simulink model "prova_kalman_09_28_BUONO"  (R2020b)
settings: Solver=ode4  StartTime=0.0  StopTime=Inf  FixedStep=0.02  RelTol=1e-3
PostLoadFcn:
  | , if any(exist('dsrtsu_mdlpostloadfcn', 'file') == [2, 3, 6]), try dsrtsu_mdlpostloadfcn('Execute', bdroot); catch fprintf('Error in PostLoadFcn (dsrtsu_mdlpostloadfcn) for model "%s":\n %s\n', bdroot, lasterr); end, end,
InitFcn:
  | , if any(exist('rtifpga_mdlclblib', 'file') ~= 0), rtifpga_mdlclblib('Init', bdroot); end,
values from neighbouring files (symbols this model uses):
  bias = [baccxINI_new,baccyINI_new,bacczINI_new,bpINI_new,bqINI_new,brINI_new]    [Loader_volo.m]
  Q1B = [    2e-15;                  2e-15 ... (first row only)    [COV_F1B_HIL.m]    (also in COV_F1B_VOLO_UP1.m = [    1.4e-14;                  1.5e-14; COV_F1B_VOLO_UP2.m = [    1.2e-14;                  1.7e-14)
  R1B = [     2e-14;                   2e-14 ... (first row only)    [COV_F1B_HIL.m]    (also in COV_F1B_VOLO_UP1.m = [     1e-13;                  1e-13; COV_F1B_VOLO_UP2.m = [     0.75e-13;                  0.9e-13)
  Sensor_Offsets = [0,0,0]    [Loader_volo.m]
  T_cal = 0.4    [Loader_volo.m]
  UP = 1    [Loader_volo.m]
  vd_ini = 0    [Loader_volo.m]
undefined symbols (not defined in the file or in its folder): DiscIntNeverNeededParam, Green, led0
libraries: simulink_extras x12, embdlinuxlib x3, raspberrypiCommlib x2, svdutilitieslib x2, aerosimlib x2, raspberrypiBasiclib x1, dspsigops x1
Description:
  | Standard RTI1006 template.
  | Supported MATLAB version:  R2020b.
settings Model: Tag=RTI1006  DSRTSU_INTERNAL_RTI_VER=570  DSRTSU_INTERNAL_RTI_TYPE=rti1006  RTICANMMDATA=struct('GeneralSetupData',struct('modelroot','C:\SUBTEAMS_2020_2021\SOFTWARE\AUTOPILOTA\drive1\Load_hardware\Raspberry_v2_1','generalsettings',struct('filesettings',struct('destfolder',struct('Name','RTICANMM_FILES','Check',1),'buildfolder',struct('Name','.','Check',1),'AbsDestfolder',struct('Name','C:\SUBTEAMS_2020_2021\SOFTWARE\AUTOPILOTA\drive1\Load_hardware\Raspberry_v2_1\RTICANMM_FILES'),'AbsBuildfolder',struct('Name','C:\SUBTEAMS_2020_2021\SOFTWARE\AUTOPILOTA\drive1\Load_hardware\Raspberry_v2_1'))),'options',struct('addpaths',1,'rmpaths',1,'addtrcexclusion',true,'cannavigator',struct('checkmonitoring',0),'show_usrtrc',0,'use_usrtrc',0),'advanced',struct('options',ones(1,100)),'MPSetup',{{}},'RTI',struct('Type','ERT','Ver','','Date',''),'modelname','prova_kalman_09_28_BUONO','block','prova_kalman_09_28_BUONO'))  DSRTSU_INTERNAL_RTIFPGA=170  Creator=lapis-dspace  LastModifiedBy=lapis-dspace
settings SolverCC: PositivePriorityOrder=on
settings DataIOCC: SaveOutput=off  SignalLogging=off  DSMLogging=off  SaveTime=off  ReturnWorkspaceOutputs=off
settings OptimizationCC: EnhancedBackFolding=on  PassReuseOutputArgsAs=Individual arguments  MaxStackSize=64  OptimizeBlockOrder=speed  DifferentSizesBufferReuse=on  OptimizationCustomize=off  EfficientTunableParamExpr=on
settings DebuggingCC: ParameterTunabilityLossMsg=error  PregeneratedLibrarySubsystemCodeDiagnostic=none  ArithmeticOperatorsInVariantConditions=warning
settings HardwareCC: ProdBitPerPointer=32  ProdBitPerSizeT=32  ProdBitPerPtrDiffT=32  ProdLargestAtomicInteger=Long  ProdLargestAtomicFloat=Double  ProdWordSize=32  ProdHWDeviceType=ARM Compatible->ARM Cortex  TargetIntDivRoundTo=Zero  TargetEndianess=LittleEndian  TargetHWDeviceType=Custom Processor->Custom
settings SFSimCC: SimUseLocalCustomCode=off  MATLABDynamicMemAlloc=off  CustomCodeUndefinedFunction=UseInterfaceOnly
settings RTWCC: Description=Embedded Coder  SystemTargetFile=ert.tlc  HardwareBoard=Raspberry Pi  TLCOptions="-aInlineSetEventsForThisBaseRateFcn=TLC_FALSE -aSuppressMultiTaskScheduler=TLC_FALSE  -aRateBasedStepFcn=0"  TemplateMakefile=ert_default_tmf  RTWUseLocalCustomCode=off  Toolchain=GNU GCC Raspberry Pi  BuildConfiguration=Faster Runs
settings CodeAppCC: ForceParamTrailComments=on  IgnoreCustomStorageClasses=off  OperatorAnnotations=on  SimulinkDataObjDesc=on  SFDataObjDesc=on  InsertBlockDesc=on
settings ERTTargetCC: MatFileLogging=on  SupportVariableSizeSignals=on
settings ConfigComp: CovMetricSettings=dswe

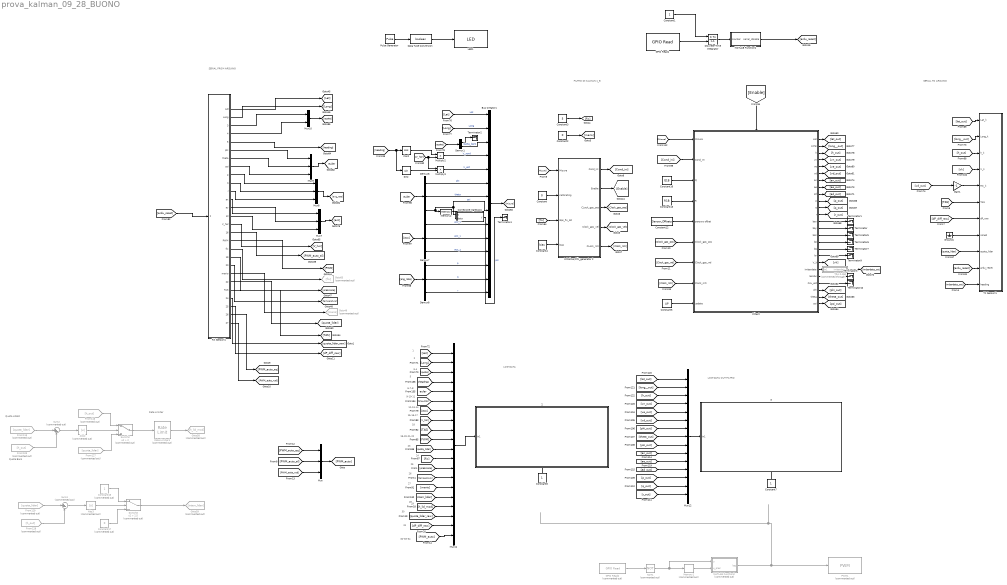
== system prova_kalman_09_28_BUONO ==
  note: 32-33-34
  note: 31
  note: 30
  note: 29
  note: 28
  note: 27
  note: 26
  note: 25
  note: 24
  note: 23
  note: 19-20-21-22
  note: 18
  note: 15-16-17
  note: 12-13-14
  note: 9-10-11
  note: 6-7-8
  note: 5
  note: 3-4
  note: 1
  note: SERIAL FROM ARDUINO
  note: LOG-DATA
  note: SERIAL TO ARDUINO
  note: LOG-DATA OUT FILTRO
  note: FILTRO DI KALMAN 1_B
  note: Rate Limiter
  note: Quota Baro
  note: Quota LIDAR
  note: 2
  " 2" : Subsystem
  " 3" : Subsystem
  Abs2 : Abs  Commented=on
  Abs3 : Abs  Commented=on
  Bus Creator1 : BusCreator  Inputs=14
  Constant : Constant  Value=0
  Constant1 : Constant  SampleTime=0.02
  Constant12 : Constant  Value=Sensor_Offsets
  Constant13 : Constant  Value=R1B
  Constant15 : Constant  Commented=on
  Constant16 : Constant  Value=Q1B
  Constant17 : Constant  Commented=on  Value=0
  Constant2 : Constant  Value=0
  Constant3 : Constant  Value=5
  Constant4 : Constant  Value=bias
  Constant5 : Constant  Value=UP
  Constant6 : Constant
  Constant7 : Constant
  Correzione ingresso1 : MATLAB Function  TreatAsAtomicUnit=on
  Cos2 : Trigonometry  Operator=cos
  Data Type Conversion : DataTypeConversion  OutDataTypeStr=boolean
  Demux1 : Demux  Outputs=2
  Demux6 : Demux  Outputs=3
  Demux7 : Demux  Outputs=3
  Demux8 : Demux  Outputs=3
  Discrete-Time Integrator : DiscreteIntegrator  ExternalReset=falling  SampleTime=0.02  LimitOutput=on  UpperSaturationLimit=1  LowerSaturationLimit=0  ICPrevOutput=DiscIntNeverNeededParam  ICPrevScaledInput=DiscIntNeverNeededParam
  Filter2 : Subsystem
  From103 : From  Commented=on  GotoTag=h_out
  From113 : From  Commented=on  GotoTag=quota_lidar
  From116 : From  Commented=on  GotoTag=h_out
  From127 : From  Commented=on  GotoTag=quota_lidar
  From128 : From  Commented=on  GotoTag=h_out
  From129 : From  Commented=on  GotoTag=quota_lidar
  GPIO Read1 : embdlinuxlib/GPIO Read  board=Pi 3 Model B  gpio=21  internalResistor=Off  sampleTime=0.02  direction=Input  blockPlatform=Raspberry Pi
      settings: SourceProductBaseCode=SC_BEAGLEBONE_BLUE,NVIDIA,RASPPI
  GPIO Read2 : embdlinuxlib/GPIO Read  Commented=on  board=Pi 3 Model B  gpio=4  internalResistor=Off  sampleTime=0.1  direction=Input  blockPlatform=Raspberry Pi
      settings: SourceProductBaseCode=SC_BEAGLEBONE_BLUE,NVIDIA,RASPPI
  Gain1 : Gain  Gain=-1
  Goto49 : Goto  Commented=on  GotoTag=mario
  Goto58 : Goto  Commented=on  GotoTag=h_lid_mod
  Goto59 : Goto  Commented=on  GotoTag=interr_lidar
  Goto83 : Goto  Commented=on  GotoTag=fix
  Ground1 : Ground
  LED1 : embdlinuxlib/LED  board=Pi 3 Model B  led=led0 (Green)  blockPlatform=Raspberry Pi
      settings: SourceProductBaseCode=SC_BEAGLEBONE_BLUE,NVIDIA,RASPPI
  MATLAB Function1 : MATLAB Function  TreatAsAtomicUnit=on
  MATLAB Function2 : MATLAB Function  Commented=on  TreatAsAtomicUnit=on
  Memory1 : Memory  Commented=on  InheritSampleTime=on
  Memory2 : Memory
  Multiply2 : Product
  Multiply3 : Product
  Mux{,7..9} (4 alike) : Mux  Inputs=3
  Mux10 : Mux  Inputs=2
  Mux11 : Mux  Inputs=20
  Mux12 : Mux  Inputs=15
  NOT1 : Logic  Commented=on  Operator=NOT  IconShape=distinctive  AllPortsSameDT=off  OutDataTypeStr=boolean
  PWM1 : raspberrypiBasiclib/PWM  Commented=on  board=Pi 3 Model B  Pin_=17  Frequency=10  blockPlatform=Raspberry Pi
      settings: SourceProductBaseCode=RASPPI
  Pulse Generator : DiscretePulseGenerator  PulseType=Time based  Period=1  PulseWidth=20
  RX Sensori1 : Subsystem
  Rate Limiter1 : RateLimiter  Commented=on  RisingSlewLimit=6  FallingSlewLimit=-6  SampleTimeMode=inherited
  Sin2 : Trigonometry
  Sum2 : Sum  Commented=on  Inputs=|+-
  Sum3 : Sum  Commented=on  Inputs=|+-
  Switch2 : Switch  Commented=on  Criteria=u2 > Threshold  Threshold=2
  Switch3 : Switch  Commented=on  Criteria=u2 > Threshold  Threshold=2.5
  TRA 0-360 : Subsystem  Commented=through
  TX Sensori1 : Subsystem
  Terminator{,1..7,9..10} (10 alike) : Terminator
  initializer/Clk_generator 2 : Subsystem
  tag scope: euler=global
  wires:
  Filter2/6(vd) -> [vd_out]
  Filter2/4(vn) -> [vn_out]
  RX Sensori1/12(ax) -> Mux7/1
  Filter2/24(theta) -> [theta_out]
  Filter2/2(Long) -> [long__out]
  Filter2/23(phi) -> [phi_out]
  Constant1/1 -> Discrete-Time Integrator/1
  RX Sensori1/11(r) -> Mux8/3
  Filter2/9(ad) -> [ad_out]
  [mario] -> Mux11/15
  TRA 0-360/1(imbardata) -> [imbardata_out]
  NOT1/1 -> MATLAB Function2/1(u), Memory1/1
  Demux7/1 -> Bus Creator1/9  "acc_x"
  RX Sensori1/18(fix) -> Goto83/1
  Multiply3/1 -> Bus Creator1/5  "V_est"
  [lat_out] -> Mux12/1
  [Lat] -> Mux11/1
  Demux7/3 -> Bus Creator1/11  "acc_z"
  Mux/1 -> [PWM_auto]
  [Cond_ini] -> Filter2/2(Cond_ini)
  Memory2/1 -> Correzione ingresso1/2(data)
  Filter2/11(q) -> [q_out]
  [PWM_auto_eq] -> Mux/1
  Filter2/25(psi) -> [psi_out]
  Discrete-Time Integrator/1 -> MATLAB Function1/1(counter)
  [PWM_auto] -> Mux11/20
  [PWM_auto_al] -> Mux/2
  [quota_lidar] -> TX Sensori1/9(quota_lidar)
  Filter2/16(bp) -> Terminator6/1
  [phi_out] -> Mux12/7
  [r_out] -> Mux12/15
  [quote] -> Demux1/1
  Filter2/20(Imbardata) -> TRA 0-360/1(In1)
  [q_out] -> Mux12/14
  Constant5/1 -> Filter2/9(update)
  initializer/Clk_generator 2/3(CLock_gps_pos) -> [Clock_gps_pos]
  initializer/Clk_generator 2/2(Enable) -> [Enable]
  [fix] -> Mux11/12
  [Clock_gps_vel] -> Filter2/7(Clock_gps_vel)
  [Clock_gps_pos] -> Filter2/6(Clock_gps_pos)
  [PWM_auto_rud] -> Mux/3
  [Long] -> Bus Creator1/2  "Long"
  Demux8/1 -> Bus Creator1/12  "p"
  RX Sensori1/26(PWM_auto_eq) -> [PWM_auto_eq]
  [Enable] -> Filter2/Enable
  Pulse Generator/1 -> Data Type Conversion/1
  Mux9/1 -> [euler]
  Filter2/22(Cov_est) -> Terminator10/1
  Demux8/2 -> Bus Creator1/13  "q"
  [ang_rate] -> Mux11/6
  [quote] -> Mux11/3
  [ardu_reset] -> TX Sensori1/10(ardu_reset)
  initializer/Clk_generator 2/1(Cond_ini) -> [Cond_ini]
  Filter2/12(r) -> [r_out]
  Constant4/1 -> initializer/Clk_generator 2/4(bias)
  Correzione ingresso1/1(y) -> Terminator4/1  "psi"
  Constant/1 -> initializer/Clk_generator 2/2(calibrating)
  initializer/Clk_generator 2/5(CLock_mti) -> [Clock_mti]
  [heading] -> Mux11/4
  Filter2/18(br) -> Terminator9/1
  Filter2/17(bq) -> Terminator7/1
  Mux12/1 -> " 3"/1(In1)
  Filter2/5(ve) -> [ve_out]
  [V_hor] -> Mux11/8
  Filter2/10(p) -> [p_out]
  [fix] -> initializer/Clk_generator 2/3(Gps_fix_3d)
  Constant3/1 -> [fix]
  Filter2/15(baz) -> Terminator5/1
  Constant2/1 -> [mario]
  Constant13/1 -> Filter2/4(R)
  RX Sensori1/5(heading) -> [heading]
  RX Sensori1/13(ay) -> Mux7/2
  Demux1/1 -> Terminator2/1
  Cos2/1 -> Multiply2/1
  Demux6/1 -> Bus Creator1/6  "phi"
  RX Sensori1/9(p) -> Mux8/1
  [ang_rate] -> Demux8/1
  RX Sensori1/2(Long) -> [Long]
  RX Sensori1/3(quota_GPS) -> Mux10/1
  [h_out] -> TX Sensori1/3(h_k)
  [acc] -> Mux11/7
  GPIO Read1/1 -> Discrete-Time Integrator/2
  Mux11/1 -> " 2"/1(In1)
  RX Sensori1/19(pressione) -> [pressione]
  [Long] -> Mux11/2
  RX Sensori1/17(PWM) -> [PWM]
  Memory1/1 -> MATLAB Function2/2(u_prec)
  Sin2/1 -> Multiply3/2
  [vd_out] -> Mux12/6
  [heading] -> Sin2/1, Cos2/1
  RX Sensori1/6(phi) -> Mux9/1
  Filter2/19(V_k) -> [vk]
  Ground1/1 -> TX Sensori1/8(none2)
  [dP_diff_raw] -> TX Sensori1/7(dP_raw)
  [an_out] -> Mux12/10
  [lat_out] -> TX Sensori1/1(Lat_k)
  [V_hor] -> Multiply3/1, Multiply2/2
  Gain1/1 -> TX Sensori1/5(RC_k)
  RX Sensori1/1(Lat) -> [Lat]
  Bus Creator1/1 -> [Misure]
  Constant16/1 -> Filter2/3(Q)
  Demux1/2 -> Bus Creator1/3  "quota_baro"
  RX Sensori1/27(PWM_auto_rud) -> [PWM_auto_rud]
  Demux7/2 -> Bus Creator1/10  "acc_y"
  RX Sensori1/14(az) -> Mux7/3
  [theta_out] -> Mux12/8
  [ve_out] -> Mux12/5
  Filter2/3(h) -> [h_out]
  Filter2/8(ae) -> [ae_out]
  Filter2/1(Lat) -> [lat_out]
  Constant12/1 -> Filter2/5(sensors offset)
  [h_out] -> Mux12/3
  Demux8/3 -> Bus Creator1/14  "r"
  MATLAB Function2/1(log) -> PWM1/1
  [imbardata_out] -> TX Sensori1/11(heading)
  [vd_out] -> Gain1/1
  Filter2/13(bax) -> Terminator1/1
  [pressione] -> Mux11/13
  Multiply2/1 -> Bus Creator1/4  "V_nord"
  [vn_out] -> Mux12/4
  RX Sensori1/20(temperatura) -> [temperatura]
  [temperatura] -> Mux11/14
  [euler] -> Demux6/1
  [p_out] -> Mux12/13
  [ardu_reset] -> RX Sensori1/1(ardu_reset)
  Filter2/21(residui) -> Terminator3/1
  RX Sensori1/4(quota_baro) -> Mux10/2
  RX Sensori1/7(theta) -> Mux9/2
  [vk] -> TX Sensori1/4(V_k)
  RX Sensori1/21(mario) -> Goto49/1
  [Clock_mti] -> Filter2/8(Clock_mti)
  [ae_out] -> Mux12/11
  RX Sensori1/16(PWM_auto_al) -> [PWM_auto_al]
  [euler] -> Mux11/5
  initializer/Clk_generator 2/4("Clock_gps_vel ") -> [Clock_gps_vel]
  Mux8/1 -> [ang_rate]
  [PWM] -> Mux11/10
  Demux6/2 -> Bus Creator1/7  "theta"
  [acc] -> Demux7/1
  Filter2/14(bay) -> Terminator/1
  [Misure] -> Filter2/1(Misure)
  [Misure] -> initializer/Clk_generator 2/1(Misure)
  [ad_out] -> Mux12/12
  Filter2/7(an) -> [an_out]
  [long__out] -> TX Sensori1/2(Long_k)
  [Lat] -> Bus Creator1/1  "Lat"
  Demux6/3 -> Memory2/1, Bus Creator1/8, Correzione ingresso1/1(u)  "psi"
  Data Type Conversion/1 -> LED1/1
  Mux7/1 -> [acc]
  RX Sensori1/8(psi) -> Mux9/3
  GPIO Read2/1 -> NOT1/1
  RX Sensori1/15(V_hor) -> [V_hor]
  [TAS] -> TX Sensori1/6(TAS)
  [psi_out] -> Mux12/9
  MATLAB Function1/1(serial_disable) -> [ardu_reset]
  Mux10/1 -> [quote]
  RX Sensori1/10(q) -> Mux8/2
  [long__out] -> Mux12/2
  Constant7/1 -> " 3"/Enable
  Constant6/1 -> " 2"/Enable
  From128/1 -> Sum3/2
  From113/1 -> Sum2/1
  Rate Limiter1/1 -> Goto58/1
  From116/1 -> Switch2/1
  From103/1 -> Sum2/2
  Constant17/1 -> Switch3/3
  From129/1 -> Sum3/1
  Sum2/1 -> Abs2/1
  Abs3/1 -> Switch3/2
  From127/1 -> Switch2/3
  Constant15/1 -> Switch3/1
  Switch2/1 -> Rate Limiter1/1
  Abs2/1 -> Switch2/2
  Sum3/1 -> Abs3/1
  Switch3/1 -> Goto59/1
  RX Sensori1/24(quota_lidar_raw) -> [quota_lidar_raw]
  RX Sensori1/23(TAS) -> [TAS]
  RX Sensori1/25(dP_diff_raw) -> [dP_diff_raw]
  RX Sensori1/22(quota_lidar) -> [quota_lidar]
  [h_lid_mod] -> Mux11/17
  [TAS] -> Mux11/9
  [dP_diff_raw] -> Mux11/19
  [interr_lidar] -> Mux11/16
  [quota_lidar] -> Mux11/11
  [quota_lidar_raw] -> Mux11/18

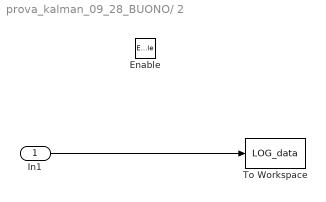
== system prova_kalman_09_28_BUONO/ 2 ==
  In1 : Inport
  Enable : EnablePort
  To Workspace : ToWorkspace  VariableName=LOG_data  SaveFormat=Structure With Time  SampleTime=0.02
  wires:
  In1/1 -> To Workspace/1

== system prova_kalman_09_28_BUONO/ 3 ==
  In1 : Inport
  Enable : EnablePort
  To Workspace : ToWorkspace  VariableName=LOG_out_filtro  SaveFormat=Structure With Time  SampleTime=0.02
  wires:
  In1/1 -> To Workspace/1

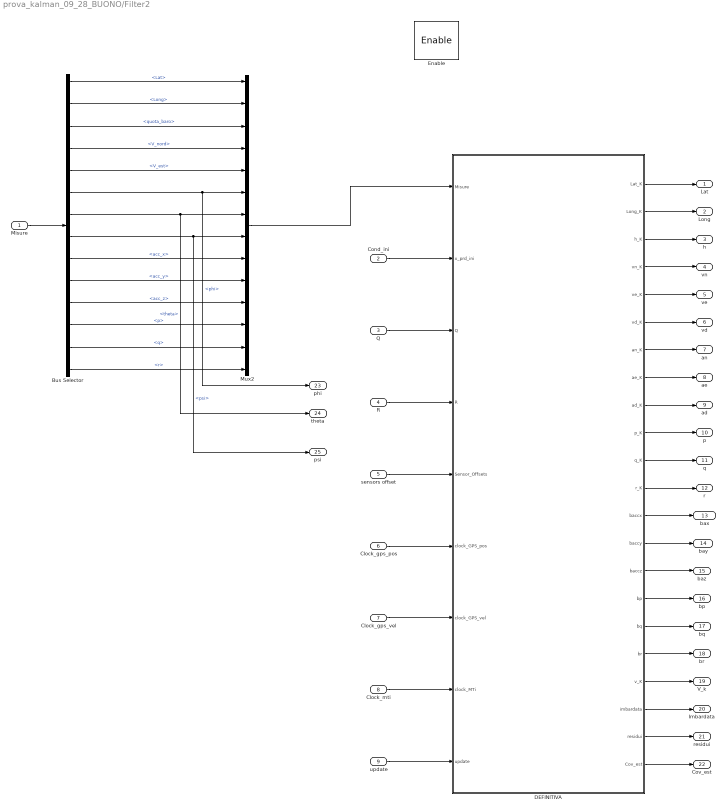
== system prova_kalman_09_28_BUONO/Filter2 ==
  Misure : Inport
  Cond_ini : Inport  Port=2
  Q : Inport  Port=3
  R : Inport  Port=4
  sensors offset : Inport  Port=5
  Clock_gps_pos : Inport  Port=6
  Clock_gps_vel : Inport  Port=7
  Clock_mti : Inport  Port=8
  update : Inport  Port=9
  Enable : EnablePort
  Bus Selector : BusSelector  OutputSignals=Lat,Long,quota_baro,V_nord,V_est,phi,theta,psi,acc_x,acc_y,acc_z,p,q,r
  DEFINITIVA : MATLAB Function  TreatAsAtomicUnit=on
  Mux2 : Mux  Inputs=14
  Lat : Outport  VectorParamsAs1DForOutWhenUnconnected=off
  Long : Outport  Port=2  VectorParamsAs1DForOutWhenUnconnected=off
  h : Outport  Port=3  VectorParamsAs1DForOutWhenUnconnected=off
  vn : Outport  Port=4  VectorParamsAs1DForOutWhenUnconnected=off
  ve : Outport  Port=5  VectorParamsAs1DForOutWhenUnconnected=off
  vd : Outport  Port=6  VectorParamsAs1DForOutWhenUnconnected=off
  an : Outport  Port=7  VectorParamsAs1DForOutWhenUnconnected=off
  ae : Outport  Port=8  VectorParamsAs1DForOutWhenUnconnected=off
  ad : Outport  Port=9  VectorParamsAs1DForOutWhenUnconnected=off
  p : Outport  Port=10  VectorParamsAs1DForOutWhenUnconnected=off
  q : Outport  Port=11  VectorParamsAs1DForOutWhenUnconnected=off
  r : Outport  Port=12  VectorParamsAs1DForOutWhenUnconnected=off
  bax : Outport  Port=13  VectorParamsAs1DForOutWhenUnconnected=off
  bay : Outport  Port=14  VectorParamsAs1DForOutWhenUnconnected=off
  baz : Outport  Port=15  VectorParamsAs1DForOutWhenUnconnected=off
  bp : Outport  Port=16  VectorParamsAs1DForOutWhenUnconnected=off
  bq : Outport  Port=17  VectorParamsAs1DForOutWhenUnconnected=off
  br : Outport  Port=18  VectorParamsAs1DForOutWhenUnconnected=off
  V_k : Outport  Port=19  VectorParamsAs1DForOutWhenUnconnected=off
  Imbardata : Outport  Port=20  VectorParamsAs1DForOutWhenUnconnected=off
  residui : Outport  Port=21  VectorParamsAs1DForOutWhenUnconnected=off
  Cov_est : Outport  Port=22  VectorParamsAs1DForOutWhenUnconnected=off
  phi : Outport  Port=23  VectorParamsAs1DForOutWhenUnconnected=off
  theta : Outport  Port=24  VectorParamsAs1DForOutWhenUnconnected=off
  psi : Outport  Port=25  VectorParamsAs1DForOutWhenUnconnected=off
  wires:
  Misure/1 -> Bus Selector/1
  Bus Selector/10 -> Mux2/10  "<acc_y>"
  Bus Selector/13 -> Mux2/13  "<q>"
  Bus Selector/11 -> Mux2/11  "<acc_z>"
  Bus Selector/4 -> Mux2/4  "<V_nord>"
  Bus Selector/14 -> Mux2/14  "<r>"
  Bus Selector/7 -> theta/1, Mux2/7  "<theta>"
  Bus Selector/12 -> Mux2/12  "<p>"
  Bus Selector/1 -> Mux2/1  "<Lat>"
  Bus Selector/6 -> phi/1, Mux2/6  "<phi>"
  Bus Selector/5 -> Mux2/5  "<V_est>"
  Bus Selector/9 -> Mux2/9  "<acc_x>"
  Bus Selector/8 -> psi/1, Mux2/8  "<psi>"
  Bus Selector/3 -> Mux2/3  "<quota_baro>"
  Bus Selector/2 -> Mux2/2  "<Long>"
  DEFINITIVA/8(ae_K) -> ae/1
  DEFINITIVA/7(an_K) -> an/1
  DEFINITIVA/11(q_K) -> q/1
  DEFINITIVA/2(Long_K) -> Long/1
  DEFINITIVA/3(h_K) -> h/1
  DEFINITIVA/10(p_K) -> p/1
  DEFINITIVA/6(vd_K) -> vd/1
  DEFINITIVA/13(baccx) -> bax/1
  DEFINITIVA/20(imbardata) -> Imbardata/1
  DEFINITIVA/19(v_K) -> V_k/1
  DEFINITIVA/18(br) -> br/1
  DEFINITIVA/4(vn_K) -> vn/1
  DEFINITIVA/16(bp) -> bp/1
  DEFINITIVA/21(residui) -> residui/1
  DEFINITIVA/17(bq) -> bq/1
  DEFINITIVA/5(ve_K) -> ve/1
  DEFINITIVA/12(r_K) -> r/1
  DEFINITIVA/1(Lat_K) -> Lat/1
  DEFINITIVA/22(Cov_est) -> Cov_est/1
  DEFINITIVA/15(baccz) -> baz/1
  DEFINITIVA/14(baccy) -> bay/1
  DEFINITIVA/9(ad_K) -> ad/1
  Mux2/1 -> DEFINITIVA/1(Misure)
  Cond_ini/1 -> DEFINITIVA/2(x_prd_ini)
  Q/1 -> DEFINITIVA/3(Q)
  R/1 -> DEFINITIVA/4(R)
  sensors offset/1 -> DEFINITIVA/5(Sensor_Offsets)
  Clock_gps_pos/1 -> DEFINITIVA/6(clock_GPS_pos)
  Clock_gps_vel/1 -> DEFINITIVA/7(clock_GPS_vel)
  Clock_mti/1 -> DEFINITIVA/8(clock_MTi)
  update/1 -> DEFINITIVA/9(update)

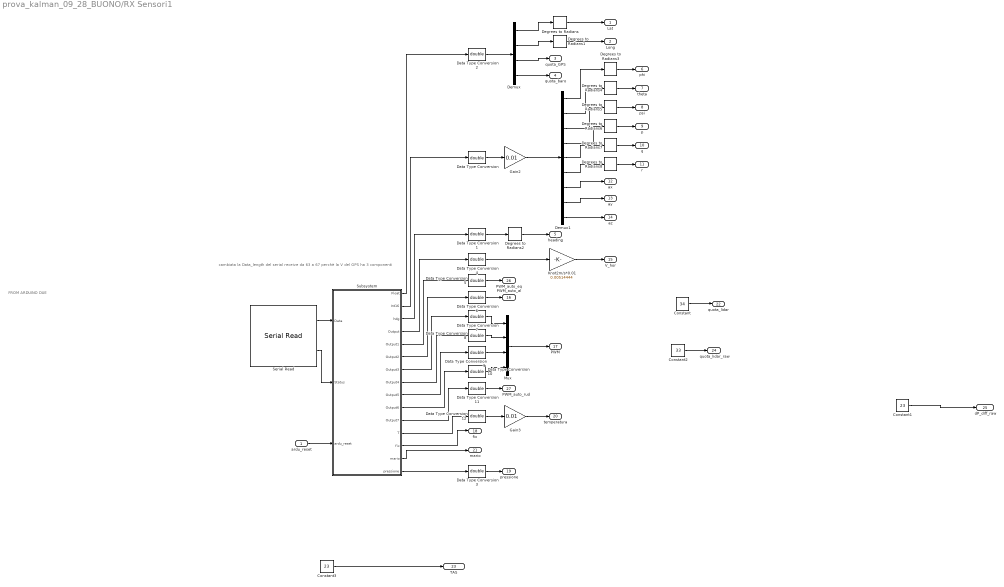
== system prova_kalman_09_28_BUONO/RX Sensori1 ==
  note: FROM ARDUINO DUE
  note: cambiata la Data_length del serial receive da 63 a 67 perchè la V del GPS ha 3 componenti
  ardu_reset : Inport
  Constant : Constant  Value=34
  Constant1 : Constant  Value=23
  Constant2 : Constant  Value=33
  Constant3 : Constant  Value=23
  Data Type Conversion{,1..12} (13 alike) : DataTypeConversion  OutDataTypeStr=double
  Degrees to Radians{,1..8} (9 alike) : simulink_extras/Transformations/Degrees to Radians
  Demux : Demux
  Demux1 : Demux  Outputs=9
  Gain2 : Gain  Gain=0.01
  Gain3 : Gain  Gain=0.01
  Knot2m/s*0.01 : Gain  Gain=0.00514444
  Mux : Mux
  Serial Read : raspberrypiCommlib/Serial Read  board=Pi 3 Model B  SCIModule_=/dev/ttyAMA0  Baudrate_=57600  Parity=None  StopBits_=1  HardwareFlowControl=None  ByteOrder=LittleEndian  DataLength=67  DataType=uint8  OutputStatus=on  SampleTime=0.02  blockPlatform=RaspberryPi
      settings: SourceProductBaseCode=RASPPI
  Subsystem : Subsystem
  Lat : Outport  VectorParamsAs1DForOutWhenUnconnected=off
  Long : Outport  Port=2  VectorParamsAs1DForOutWhenUnconnected=off
  quota_GPS : Outport  Port=3  VectorParamsAs1DForOutWhenUnconnected=off
  quota_baro : Outport  Port=4  VectorParamsAs1DForOutWhenUnconnected=off
  heading : Outport  Port=5  VectorParamsAs1DForOutWhenUnconnected=off
  phi : Outport  Port=6  VectorParamsAs1DForOutWhenUnconnected=off
  theta : Outport  Port=7  VectorParamsAs1DForOutWhenUnconnected=off
  psi : Outport  Port=8  VectorParamsAs1DForOutWhenUnconnected=off
  p : Outport  Port=9  VectorParamsAs1DForOutWhenUnconnected=off
  q : Outport  Port=10  VectorParamsAs1DForOutWhenUnconnected=off
  r : Outport  Port=11  VectorParamsAs1DForOutWhenUnconnected=off
  ax : Outport  Port=12  VectorParamsAs1DForOutWhenUnconnected=off
  ay : Outport  Port=13  VectorParamsAs1DForOutWhenUnconnected=off
  az : Outport  Port=14  VectorParamsAs1DForOutWhenUnconnected=off
  V_hor : Outport  Port=15  VectorParamsAs1DForOutWhenUnconnected=off
  PWM_auto_al : Outport  Port=16  VectorParamsAs1DForOutWhenUnconnected=off
  PWM : Outport  Port=17  VectorParamsAs1DForOutWhenUnconnected=off
  fix : Outport  Port=18  VectorParamsAs1DForOutWhenUnconnected=off
  pressione : Outport  Port=19  VectorParamsAs1DForOutWhenUnconnected=off
  temperatura : Outport  Port=20  VectorParamsAs1DForOutWhenUnconnected=off
  mario : Outport  Port=21  OutDataTypeStr=double  VectorParamsAs1DForOutWhenUnconnected=off
  quota_lidar : Outport  Port=22
  TAS : Outport  Port=23
  quota_lidar_raw : Outport  Port=24
  dP_diff_raw : Outport  Port=25
  PWM_auto_eq : Outport  Port=26  VectorParamsAs1DForOutWhenUnconnected=off
  PWM_auto_rud : Outport  Port=27  VectorParamsAs1DForOutWhenUnconnected=off
  wires:
  Data Type Conversion12/1 -> Gain3/1
  Subsystem/3(hdg) -> Data Type Conversion1/1
  Subsystem/11(Output7) -> Data Type Conversion11/1
  Subsystem/15(pressione) -> Data Type Conversion3/1
  Degrees to Radians1/1 -> Long/1
  Subsystem/10(Output6) -> Data Type Conversion10/1
  Data Type Conversion1/1 -> Degrees to Radians2/1
  Subsystem/1(Float) -> Data Type Conversion2/1
  Demux/4 -> quota_baro/1
  Subsystem/5(Output1) -> Data Type Conversion5/1
  Data Type Conversion11/1 -> PWM_auto_rud/1
  Data Type Conversion10/1 -> Mux/4
  Data Type Conversion9/1 -> Mux/3
  Demux1/2 -> Degrees to Radians4/1
  Degrees to Radians6/1 -> p/1
  Demux1/4 -> Degrees to Radians6/1
  Subsystem/6(Output2) -> Data Type Conversion6/1
  Subsystem/8(Output4) -> Data Type Conversion8/1
  Degrees to Radians5/1 -> psi/1
  Mux/1 -> PWM/1
  Demux/2 -> Degrees to Radians1/1
  Subsystem/2(Int16) -> Data Type Conversion/1
  Subsystem/9(Output5) -> Data Type Conversion9/1
  Data Type Conversion2/1 -> Demux/1
  Subsystem/7(Output3) -> Data Type Conversion7/1
  Demux1/1 -> Degrees to Radians3/1
  Demux1/9 -> az/1
  Subsystem/4(Output) -> Data Type Conversion4/1
  Gain2/1 -> Demux1/1
  Demux1/7 -> ax/1
  Data Type Conversion6/1 -> PWM_auto_al/1
  Data Type Conversion3/1 -> pressione/1
  Subsystem/14(mario) -> mario/1
  Degrees to Radians7/1 -> q/1
  Subsystem/12(T) -> Data Type Conversion12/1
  Serial Read/1 -> Subsystem/1(Data)
  Serial Read/2 -> Subsystem/2(Status)
  Gain3/1 -> temperatura/1
  Degrees to Radians8/1 -> r/1
  Degrees to Radians/1 -> Lat/1
  ardu_reset/1 -> Subsystem/3(ardu_reset)
  Demux1/8 -> ay/1
  Data Type Conversion8/1 -> Mux/2
  Degrees to Radians4/1 -> theta/1
  Demux1/5 -> Degrees to Radians7/1
  Subsystem/13(fix) -> fix/1
  Data Type Conversion/1 -> Gain2/1
  Degrees to Radians3/1 -> phi/1
  Knot2m/s*0.01/1 -> V_hor/1
  Demux/1 -> Degrees to Radians/1
  Data Type Conversion4/1 -> Knot2m/s*0.01/1
  Data Type Conversion7/1 -> Mux/1
  Data Type Conversion5/1 -> PWM_auto_eq/1
  Demux/3 -> quota_GPS/1
  Demux1/3 -> Degrees to Radians5/1
  Demux1/6 -> Degrees to Radians8/1
  Degrees to Radians2/1 -> heading/1
  Constant1/1 -> dP_diff_raw/1
  Constant2/1 -> quota_lidar_raw/1
  Constant/1 -> quota_lidar/1
  Constant3/1 -> TAS/1

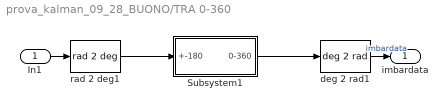
== system prova_kalman_09_28_BUONO/TRA 0-360 ==
  In1 : Inport
  Subsystem1 : Subsystem
  deg 2 rad1 : aerosimlib/Unit Conversion/Angular position/deg 2 rad
      settings: SourceProductName=AeroSim Blockset
  rad 2 deg1 : aerosimlib/Unit Conversion/Angular position/rad 2 deg
      settings: SourceProductName=AeroSim Blockset
  imbardata : Outport  VectorParamsAs1DForOutWhenUnconnected=off
  wires:
  deg 2 rad1/1 -> imbardata/1  "imbardata"
  rad 2 deg1/1 -> Subsystem1/1(+-180)
  In1/1 -> rad 2 deg1/1
  Subsystem1/1(0-360) -> deg 2 rad1/1

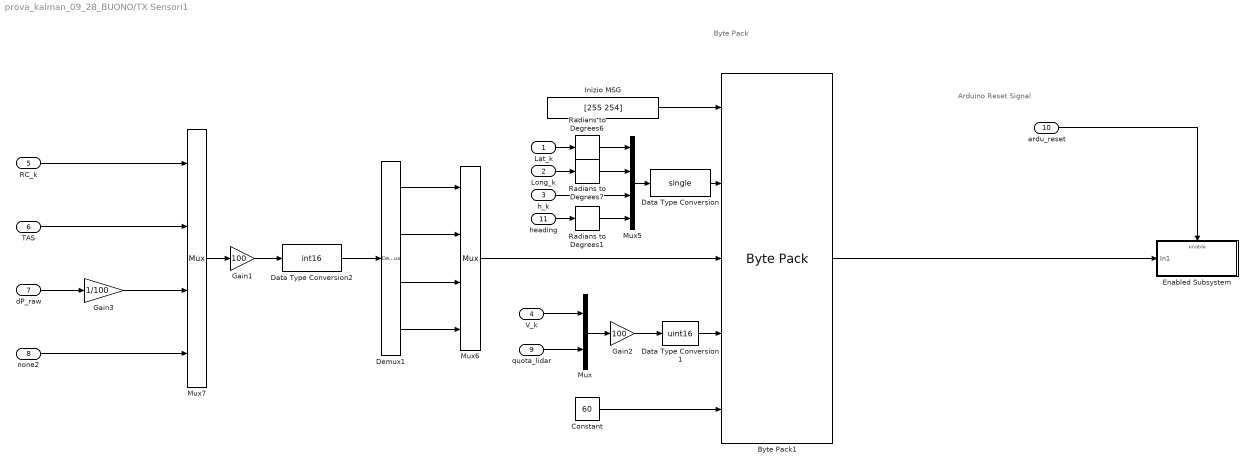
== system prova_kalman_09_28_BUONO/TX Sensori1 ==
  note: Byte Pack
  note: Arduino Reset Signal
  Lat_k : Inport
  Long_k : Inport  Port=2
  h_k : Inport  Port=3
  V_k : Inport  Port=4
  RC_k : Inport  Port=5
  TAS : Inport  Port=6
  dP_raw : Inport  Port=7
  none2 : Inport  Port=8
  quota_lidar : Inport  Port=9
  ardu_reset : Inport  Port=10
  heading : Inport  Port=11
  Byte Pack1 : svdutilitieslib/Byte Pack  maskPackedDataType=uint8  datatypes={'uint8','single','int16','uint16','uint8'}  byteAlign=1  blockPlatform=arduinoert
      settings: SourceProductBaseCode=ANDROID,ARDUINO,ML_ARDUINO,ECCORTEXA,ECCORTEXR,SC_BEAGLEBONE_BLUE,EC_FREEDOM_BOARD,EC_FRDM_K64F,INTEL_BLOCKSET,JETSONCPU,MICROBIT,NUCLEO,NVIDIA,PX4AUTOPILOTS,RASPPIIO,STMICRODIS,TIC2000,XILINX_BLOCKSET
  Constant : Constant  Value=60  OutDataTypeStr=uint8
  Data Type Conversion : DataTypeConversion  OutDataTypeStr=single
  Data Type Conversion1 : DataTypeConversion  OutDataTypeStr=uint16
  Data Type Conversion2 : DataTypeConversion  OutDataTypeStr=int16
  Demux1 : Demux
  Enabled Subsystem : Subsystem  TreatAsAtomicUnit=on
  Gain1 : Gain  Gain=100
  Gain2 : Gain  Gain=100
  Gain3 : Gain  Gain=1/100
  Inizio MSG : Constant  Value=[255 254]  OutDataTypeStr=uint8  SampleTime=0.02
  Mux : Mux  Inputs=2
  Mux5 : Mux
  Mux6 : Mux
  Mux7 : Mux
  Radians to Degrees1 : simulink_extras/Transformations/Radians to Degrees
  Radians to Degrees6 : simulink_extras/Transformations/Radians to Degrees
  Radians to Degrees7 : simulink_extras/Transformations/Radians to Degrees
  wires:
  h_k/1 -> Mux5/3
  Gain1/1 -> Data Type Conversion2/1
  Long_k/1 -> Radians to Degrees7/1
  Demux1/4 -> Mux6/4
  Inizio MSG/1 -> Byte Pack1/1
  Demux1/1 -> Mux6/1
  Data Type Conversion2/1 -> Demux1/1
  Demux1/3 -> Mux6/3
  Byte Pack1/1 -> Enabled Subsystem/1(In1)
  Lat_k/1 -> Radians to Degrees6/1
  Mux7/1 -> Gain1/1
  Mux6/1 -> Byte Pack1/3
  Demux1/2 -> Mux6/2
  RC_k/1 -> Mux7/1
  Data Type Conversion1/1 -> Byte Pack1/4
  Gain2/1 -> Data Type Conversion1/1
  V_k/1 -> Mux/1
  Mux5/1 -> Data Type Conversion/1
  Data Type Conversion/1 -> Byte Pack1/2
  TAS/1 -> Mux7/2
  dP_raw/1 -> Gain3/1
  none2/1 -> Mux7/4
  Radians to Degrees6/1 -> Mux5/1
  Radians to Degrees7/1 -> Mux5/2
  ardu_reset/1 -> Enabled Subsystem/Enable
  Constant/1 -> Byte Pack1/5
  quota_lidar/1 -> Mux/2
  Mux/1 -> Gain2/1
  heading/1 -> Radians to Degrees1/1
  Radians to Degrees1/1 -> Mux5/4
  Gain3/1 -> Mux7/3

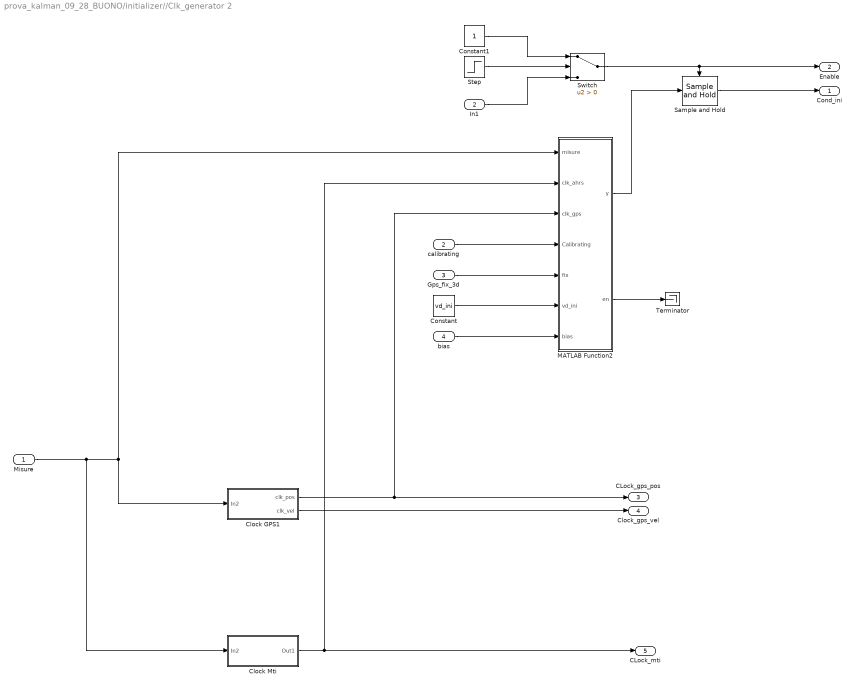
== system prova_kalman_09_28_BUONO/initializer//Clk_generator 2 ==
  Misure : Inport
  calibrating : Inport  Port=2
  Gps_fix_3d : Inport  Port=3
  bias : Inport  Port=4
  Clock GPS1 : Subsystem
  Clock Mti : Subsystem
  Constant : Constant  Value=vd_ini
  Constant1 : Constant
  In1 : InportShadow  Port=2
  MATLAB Function2 : MATLAB Function  TreatAsAtomicUnit=on
  Sample and Hold : dspsigops/Sample and Hold  trig=Rising edge  initCond=0  latchinput=off
  Step : Step  Time=T_cal  SampleTime=0.02
  Switch : Switch  Criteria=u2 > Threshold
  Terminator : Terminator
  Cond_ini : Outport  VectorParamsAs1DForOutWhenUnconnected=off
  Enable : Outport  Port=2  VectorParamsAs1DForOutWhenUnconnected=off
  CLock_gps_pos : Outport  Port=3  VectorParamsAs1DForOutWhenUnconnected=off
  "Clock_gps_vel " : Outport  Port=4  VectorParamsAs1DForOutWhenUnconnected=off
  CLock_mti : Outport  Port=5  VectorParamsAs1DForOutWhenUnconnected=off
  wires:
  Gps_fix_3d/1 -> MATLAB Function2/5(fix)
  Clock GPS1/1(clk_pos) -> MATLAB Function2/3(clk_gps), CLock_gps_pos/1
  Clock Mti/1(Out1) -> CLock_mti/1, MATLAB Function2/2(clk_ahrs)
  Constant/1 -> MATLAB Function2/6(vd_ini)
  bias/1 -> MATLAB Function2/7(bias)
  calibrating/1 -> MATLAB Function2/4(Calibrating)
  Step/1 -> Switch/2
  In1/1 -> Switch/3
  Constant1/1 -> Switch/1
  Switch/1 -> Sample and Hold/Trigger, Enable/1
  Misure/1 -> Clock Mti/1(In2), Clock GPS1/1(In2), MATLAB Function2/1(misure)
  Clock GPS1/2(clk_vel) -> "Clock_gps_vel "/1
  MATLAB Function2/1(y) -> Sample and Hold/1
  Sample and Hold/1 -> Cond_ini/1
  MATLAB Function2/2(en) -> Terminator/1

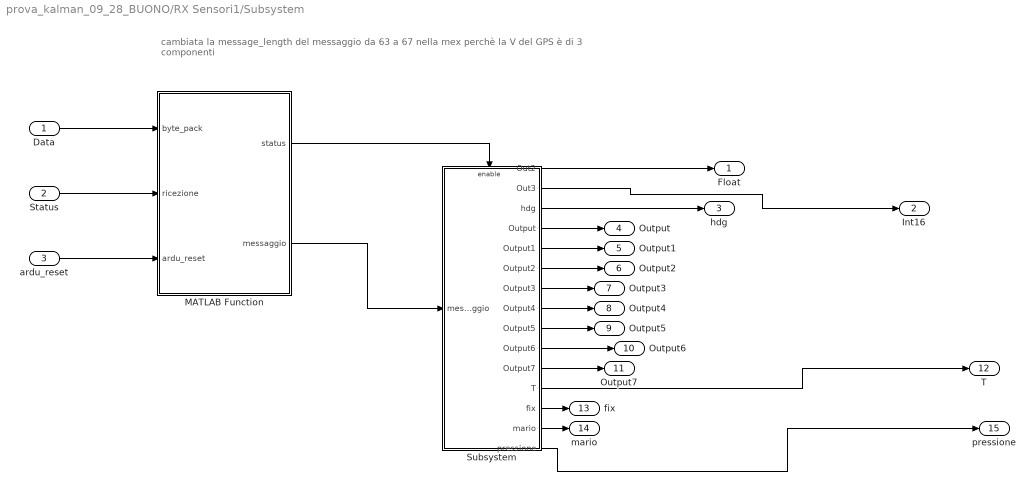
== system prova_kalman_09_28_BUONO/RX Sensori1/Subsystem ==
  note: cambiata la message_length del messaggio da 63 a 67 nella mex perchè la V del GPS è di 3 componenti
  Data : Inport
  Status : Inport  Port=2
  ardu_reset : Inport  Port=3
  MATLAB Function : MATLAB Function  TreatAsAtomicUnit=on
  Subsystem : Subsystem
  Float : Outport  VectorParamsAs1DForOutWhenUnconnected=off
  Int16 : Outport  Port=2  VectorParamsAs1DForOutWhenUnconnected=off
  hdg : Outport  Port=3  VectorParamsAs1DForOutWhenUnconnected=off
  Output : Outport  Port=4
  Output1 : Outport  Port=5
  Output2 : Outport  Port=6
  Output3 : Outport  Port=7
  Output4 : Outport  Port=8
  Output5 : Outport  Port=9
  Output6 : Outport  Port=10
  Output7 : Outport  Port=11
  T : Outport  Port=12
  fix : Outport  Port=13  VectorParamsAs1DForOutWhenUnconnected=off
  mario : Outport  Port=14  VectorParamsAs1DForOutWhenUnconnected=off
  pressione : Outport  Port=15  VectorParamsAs1DForOutWhenUnconnected=off
  wires:
  Subsystem/1(Out2) -> Float/1
  Subsystem/2(Out3) -> Int16/1
  Subsystem/3(hdg) -> hdg/1
  MATLAB Function/1(status) -> Subsystem/Enable
  MATLAB Function/2(messaggio) -> Subsystem/1(messaggio)
  Data/1 -> MATLAB Function/1(byte_pack)
  Status/1 -> MATLAB Function/2(ricezione)
  Subsystem/13("fix ") -> fix/1
  Subsystem/14(mario) -> mario/1
  Subsystem/15(pressione) -> pressione/1
  ardu_reset/1 -> MATLAB Function/3(ardu_reset)
  Subsystem/4(Output) -> Output/1
  Subsystem/5(Output1) -> Output1/1
  Subsystem/6(Output2) -> Output2/1
  Subsystem/7(Output3) -> Output3/1
  Subsystem/8(Output4) -> Output4/1
  Subsystem/9(Output5) -> Output5/1
  Subsystem/10(Output6) -> Output6/1
  Subsystem/11(Output7) -> Output7/1
  Subsystem/12(T) -> T/1

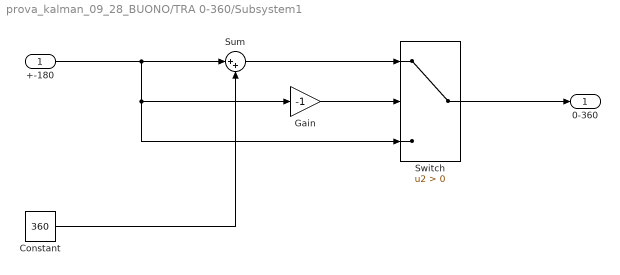
== system prova_kalman_09_28_BUONO/TRA 0-360/Subsystem1 ==
  +-180 : Inport
  Constant : Constant  Value=360
  Gain : Gain  Gain=-1
  Sum : Sum  Inputs=|++
  Switch : Switch  Criteria=u2 > Threshold
  0-360 : Outport  VectorParamsAs1DForOutWhenUnconnected=off
  wires:
  Constant/1 -> Sum/2
  +-180/1 -> Gain/1, Switch/3, Sum/1
  Gain/1 -> Switch/2
  Sum/1 -> Switch/1
  Switch/1 -> 0-360/1

== system prova_kalman_09_28_BUONO/TX Sensori1/Enabled Subsystem ==
  In1 : Inport
  Enable : EnablePort
  Serial Write : raspberrypiCommlib/Serial Write  board=Pi 3 Model B  SCIModule_=/dev/ttyAMA0  Baudrate_=57600  Parity=None  StopBits_=1  HardwareFlowControl=None  ByteOrder=LittleEndian  OutputStatus=off  blockPlatform=RaspberryPi
      settings: SourceProductBaseCode=RASPPI
  wires:
  In1/1 -> Serial Write/1

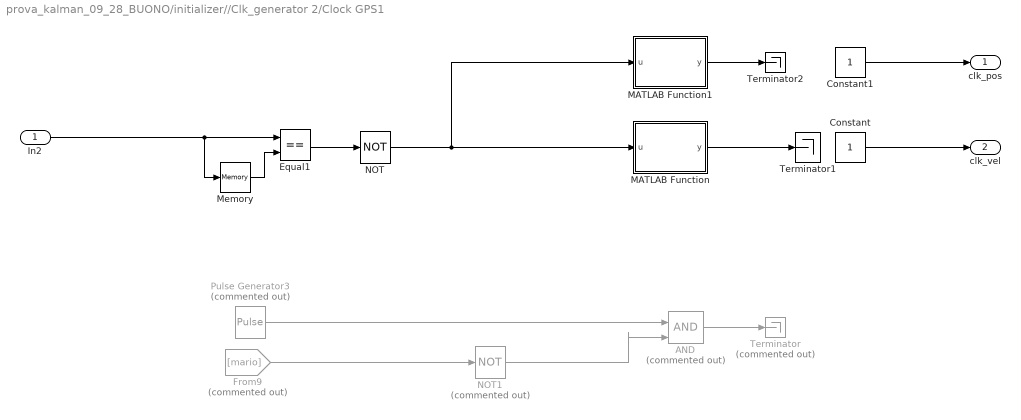
== system prova_kalman_09_28_BUONO/initializer//Clk_generator 2/Clock GPS1 ==
  In2 : Inport
  AND : Logic  Commented=on  IconShape=distinctive  AllPortsSameDT=off  OutDataTypeStr=boolean
  Constant : Constant
  Constant1 : Constant
  Equal1 : RelationalOperator  Operator===  OutDataTypeStr=boolean  RndMeth=Simplest
  From9 : From  Commented=on  GotoTag=mario
  MATLAB Function : MATLAB Function  TreatAsAtomicUnit=on
  MATLAB Function1 : MATLAB Function  TreatAsAtomicUnit=on
  Memory : Memory
  NOT : Logic  Operator=NOT  IconShape=distinctive  AllPortsSameDT=off  OutDataTypeStr=boolean
  NOT1 : Logic  Commented=on  Operator=NOT  IconShape=distinctive  AllPortsSameDT=off  OutDataTypeStr=boolean
  Pulse Generator3 : DiscretePulseGenerator  Commented=on  PulseType=Time based  Period=0.2  PulseWidth=10
  Terminator : Terminator  Commented=on
  Terminator1 : Terminator
  Terminator2 : Terminator
  clk_pos : Outport  VectorParamsAs1DForOutWhenUnconnected=off
  clk_vel : Outport  Port=2  VectorParamsAs1DForOutWhenUnconnected=off
  wires:
  Equal1/1 -> NOT/1
  NOT/1 -> MATLAB Function1/1(u), MATLAB Function/1(u)
  In2/1 -> Equal1/1, Memory/1
  Memory/1 -> Equal1/2
  From9/1 -> NOT1/1
  Pulse Generator3/1 -> AND/1
  NOT1/1 -> AND/2
  AND/1 -> Terminator/1
  MATLAB Function1/1(y) -> Terminator2/1
  MATLAB Function/1(y) -> Terminator1/1
  Constant1/1 -> clk_pos/1
  Constant/1 -> clk_vel/1

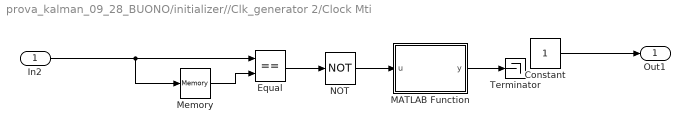
== system prova_kalman_09_28_BUONO/initializer//Clk_generator 2/Clock Mti ==
  In2 : Inport
  Constant : Constant
  Equal : RelationalOperator  Operator===  OutDataTypeStr=boolean  RndMeth=Simplest
  MATLAB Function : MATLAB Function  TreatAsAtomicUnit=on
  Memory : Memory
  NOT : Logic  Operator=NOT  IconShape=distinctive  AllPortsSameDT=off  OutDataTypeStr=boolean
  Terminator : Terminator
  Out1 : Outport  VectorParamsAs1DForOutWhenUnconnected=off
  wires:
  In2/1 -> Memory/1, Equal/1
  Equal/1 -> NOT/1
  Memory/1 -> Equal/2
  MATLAB Function/1(y) -> Terminator/1
  NOT/1 -> MATLAB Function/1(u)
  Constant/1 -> Out1/1

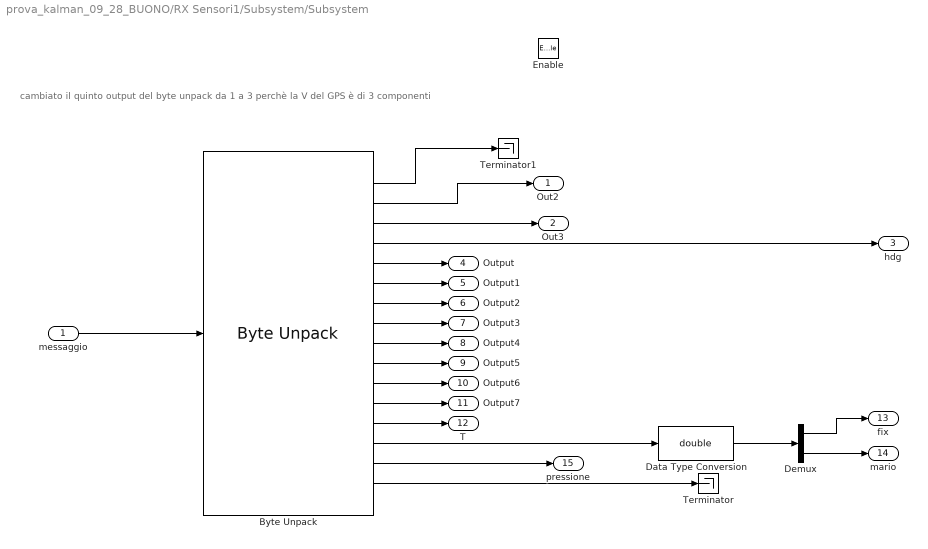
== system prova_kalman_09_28_BUONO/RX Sensori1/Subsystem/Subsystem ==
  note: cambiato il quinto output del byte unpack da 1 a 3 perchè la V del GPS è di 3 componenti
  messaggio : Inport
  Enable : EnablePort
  Byte Unpack : svdutilitieslib/Byte Unpack  dimensions={[2],[4],[9],[1],[3],[1],[1],[1],[1],[1],[1],[1],[1],[2],[1],[1]}  datatypes={'uint8','single','int16','uint16','uint16','uint16','uint16','uint16','uint16','uint16','uint16','uint16','uint16','uint8','uint32','uint8'}  byteAlign=1  blockPlatform=arduinoert
      settings: SourceProductBaseCode=ARDUINO
  Data Type Conversion : DataTypeConversion  OutDataTypeStr=double
  Demux : Demux  Outputs=2
  Terminator : Terminator
  Terminator1 : Terminator
  Out2 : Outport  VectorParamsAs1DForOutWhenUnconnected=off
  Out3 : Outport  Port=2  VectorParamsAs1DForOutWhenUnconnected=off
  hdg : Outport  Port=3  VectorParamsAs1DForOutWhenUnconnected=off
  Output : Outport  Port=4
  Output1 : Outport  Port=5
  Output2 : Outport  Port=6
  Output3 : Outport  Port=7
  Output4 : Outport  Port=8
  Output5 : Outport  Port=9
  Output6 : Outport  Port=10
  Output7 : Outport  Port=11
  T : Outport  Port=12
  "fix " : Outport  Port=13  VectorParamsAs1DForOutWhenUnconnected=off
  mario : Outport  Port=14  VectorParamsAs1DForOutWhenUnconnected=off
  pressione : Outport  Port=15  VectorParamsAs1DForOutWhenUnconnected=off
  wires:
  messaggio/1 -> Byte Unpack/1
  Byte Unpack/1 -> Terminator1/1
  Byte Unpack/4 -> hdg/1
  Byte Unpack/3 -> Out3/1
  Byte Unpack/2 -> Out2/1
  Byte Unpack/16 -> Terminator/1
  Byte Unpack/14 -> Data Type Conversion/1
  Demux/1 -> "fix "/1
  Demux/2 -> mario/1
  Data Type Conversion/1 -> Demux/1
  Byte Unpack/15 -> pressione/1
  Byte Unpack/5 -> Output/1
  Byte Unpack/6 -> Output1/1
  Byte Unpack/7 -> Output2/1
  Byte Unpack/8 -> Output3/1
  Byte Unpack/9 -> Output4/1
  Byte Unpack/10 -> Output5/1
  Byte Unpack/11 -> Output6/1
  Byte Unpack/12 -> Output7/1
  Byte Unpack/13 -> T/1

== matlab function prova_kalman_09_28_BUONO/initializer//Clk_generator 2/Clock GPS1/MATLAB Function ==
  data: u input; y output
function y = fcn(u)

 y = u(4) || u(5);

% if mario ~=0
%     
%     y=double(0);
%     
% else 
%      y = u(1) || u(2) || u(3) || u(4);
% 
%  end

== matlab function prova_kalman_09_28_BUONO/initializer//Clk_generator 2/Clock GPS1/MATLAB Function1 ==
  data: u input; y output
function y = fcn(u)

 y = u(1) || u(2);
% if mario ~=0
%     
%     y=double(0);
%     
% else 
%      y = u(1) || u(2) || u(3) || u(4);
% 
%  end

== matlab function prova_kalman_09_28_BUONO/MATLAB Function1 ==
  data: counter input; serial_disable output
function serial_disable = fcn(counter)

if counter < 1
    serial_disable = 0;
else
    serial_disable = 1;
end

== matlab function prova_kalman_09_28_BUONO/initializer//Clk_generator 2/MATLAB Function2 ==
  data: misure input; clk_ahrs input; y output; clk_gps input; Calibrating input; en output; fix input; vd_ini input; bias input
function [y,en] = fcn(misure,clk_ahrs,clk_gps,Calibrating, fix,vd_ini, bias)

     y=zeros(21,1);
    
     phi = misure(6);
     theta = misure(7);
     psi = misure(8);
    
     ab=[misure(9);misure(10);misure(11)];
     
     
    LBE= [cos(psi)*cos(theta) ,cos(psi)*sin(phi)*sin(theta)-cos(phi)*sin(psi) ,cos(phi)*cos(psi)*sin(theta)+sin(phi)*sin(psi);
    
      sin(psi)*cos(theta) ,sin(phi)*sin(psi)*sin(theta)+cos(phi)*cos(psi) , cos(phi)*sin(psi)*sin(theta)-cos(psi)*sin(phi);
      
      -sin(theta),cos(theta)*sin(phi),cos(phi)*cos(theta)];
      
      aterra=LBE*ab;
   
    
    y(1) = misure(1);
    y(2) = misure(2);
    y(3) = misure(3);
    
    
    y(4) = misure(4);
    y(5) = misure(5);
    y(6) = vd_ini;
    
    y(7) = misure(6);
    y(8) = misure(7);
    y(9) = misure(8);
    
    y(10) = aterra(1);
    y(11) = aterra(2);
    y(12) = aterra(3);
    
    y(13) = misure(12);
    y(14) = misure(13);
    y(15) = misure(14);
    
    y(16) = bias(1);
    y(17) = bias(2);
    y(18) = bias(3);
    
    y(19) = bias(4);
    y(20) = bias(5);
    y(21) = bias(6);
    
    
en=1;

== matlab function prova_kalman_09_28_BUONO/MATLAB Function2 ==
  data: u input; log output; u_prec input
function log = fcn(u,u_prec)

persistent  status spento

if isempty(status) 
    status = 0 ;
end
if isempty(spento) 
    spento = true ;
end

if (u == 1 && u_prec == 0 )
    if spento == true 
        status = 1  ;  
        spento = false ;
    else 
        status = 0 ;
        spento = true ;
    end
end

% if status == 1 && ( u == 0 && u_prec == 1 )
%     
% end
    



log = status  ;
end

== matlab function prova_kalman_09_28_BUONO/RX Sensori1/Subsystem/MATLAB Function ==
  data: byte_pack input; status output; messaggio output; ricezione input; ardu_reset input
function [status,messaggio]  = LETTURA_Arduino_mex(byte_pack,ricezione,ardu_reset)

persistent message counter start_found

message_length=67; %%cambiato da 63 a 67

status = false;                                        %ho aggiunto questo
messaggio = uint8(zeros(1,message_length)) ;
M = uint8(length(byte_pack)) ;
entrata = true ;

if isempty(start_found) 
     start_found = false ;
end 
if isempty (counter) 
    counter = uint8(0) ;
end 
if isempty(message)
     message = uint8(zeros(1,message_length)) ;
end

if ((ricezione ~= 0) || (ardu_reset == 0))
    start_found = false ;
    message = uint8(zeros(1,message_length)) ;
    counter = uint8(0)  ;
    entrata = false ;
end

if (start_found == 0 && entrata == true )
    for i = 1 : M-1  
        if ( byte_pack(i) == 62 &&  byte_pack(i + 1) == 255 )                  % mi conviene mandare un secondo byte all'inizio cosi non devo cambiare nulla
            message(1:M - (i-1)) = byte_pack(i:end) ;
            counter = M - (i-1) ; 
            start_found = true ;
            break
        end
    end   % lho messo qua
        if counter == M 
            messaggio = message ;
            message = uint8(zeros(1,message_length)) ;
            status = true ;
            start_found = false ;
            counter = uint8(0) ;
        end
     %end
    
    
elseif start_found == 1 

        message(counter + 1 : end) = byte_pack(1:M - counter) ;
        status = true;       %ho aggiunto questo
        messaggio = message ;
        counter = M - counter ;
        message = uint8(zeros(1,message_length)) ;
        
            for i = counter : M-1  
        if ( byte_pack(i) == 62 &&  byte_pack(i + 1) == 255 )                  % mi conviene mandare un secondo byte all'inizio cosi non devo cambiare nulla
            message(1:M - (i-1)) = byte_pack(i:end) ;
            counter = M - (i-1) ; 
            start_found = true ;
            break
        else 
            start_found = false ;
            counter = uint8(0);
        end 
            end
        
     %   message (1 : M-counter ) = byte_pack(counter + 1:end) ;
     %   counter = M - counter ;

end

== matlab function prova_kalman_09_28_BUONO/Filter2/DEFINITIVA ==
  settings: updateMethod=DISCRETE  sampleTime=0.02
  data: Lat_K output; Misure input; x_prd_ini input; Q input; R input; Sensor_Offsets input; clock_GPS_pos input; clock_GPS_vel input; clock_MTi input; Long_K output; h_K output; vn_K output; ve_K output; vd_K output; an_K output; ae_K output; ad_K output; p_K output; q_K output; r_K output; baccx output; baccy output; baccz output; bp output; bq output; br output; v_K output; imbardata output; residui output; update input; Cov_est output
function [Lat_K,Long_K,h_K,vn_K,ve_K,vd_K,an_K,ae_K,ad_K,p_K,q_K,r_K,baccx,baccy,baccz,bp,bq,br,v_K,imbardata,residui,Cov_est]     = FILTRO_1B(Misure,x_prd_ini,Q,R,Sensor_Offsets,clock_GPS_pos,clock_GPS_vel,clock_MTi,update)

persistent x_prd
persistent p_prd

%% Parametri

a = 6378137; % earth radius (m)
g = 9.81;      % gravity constant (m/s^2)

Z = Misure;
EULERO=[Z(6),Z(7),Z(8)];
% Z(9)=-Misure(9);

infinito = 1e40;

dt=0.02; %sample time

%      Sensor Offsets     %% Da spostere in avvio simulazione

rx = Sensor_Offsets(1);

ry = Sensor_Offsets(2);

rz =Sensor_Offsets(3);

% Inizializzo stato e covarianza

% if isempty(x_prd)
%
%     x_prd = x_prd_ini;
%
%  	p_prd =zeros(18,18);
%
% end




if isempty(x_prd)
    x_prd=zeros(1,18);
    
    x_prd(1) = x_prd_ini(1); %Posizione
    x_prd(2) = x_prd_ini(2);
    x_prd(3) = x_prd_ini(3);
    
    x_prd(4) = x_prd_ini(4); %Velocità
    x_prd(5) = x_prd_ini(5);
    x_prd(6) = x_prd_ini(6);
    
    x_prd(7) = x_prd_ini(10); %Acc
    x_prd(8) = x_prd_ini(11);
    x_prd(9)= x_prd_ini(12);
    
    x_prd(10) = x_prd_ini(13); %V ang
    x_prd(11) = x_prd_ini(14);
    x_prd(12)=  x_prd_ini(15);
    
    x_prd(13) = x_prd_ini(16); %Bias Acc
    x_prd(14) = x_prd_ini(17);
    x_prd(15)=  x_prd_ini(18);
    
    %      x_prd(13) =0; %Bias Acc
    %      x_prd(14) = 0;
    %      x_prd(15)=  0;
    
    
    x_prd(16) = x_prd_ini(19); %Bias Vang
    x_prd(17) = x_prd_ini(20);
    x_prd(18)=  x_prd_ini(21);
    %      x_prd(16) = 0; %Bias Vang
    %      x_prd(17) = 0;
    %      x_prd(18)=  0;
    
    %  	p_prd =10000*eye(18,18);
    p_prd =zeros(18,18);
    p_prd(1,1)=10000000000;
    p_prd(4,4)=10000000000;
    p_prd(5,5)=10000000000;
end

%%%%%%%%%%%%%%%%%%%%%%%%%%%
%% Predicted measurement %%
%%SONO LE EQUAZIONI DELLE EVOLUZIONI DELLE MISURE


Y_prd = measure_F1B(x_prd,EULERO,rx,ry,rz,g);


%%%%%%%%%%%%%%%%%%%%%%%%%%%
%% Linearize measurement-jacobiano delle equazioni delle misure%%
%%%%%%%%%%%%%%%%%%%%%%%%%%%

H=jac_H_F1B(x_prd,EULERO,rx,ry,rz,g);


%%%%%%%%%%%%%%%%%%%%%%%%
%% aggiornamento della misura %%
%%%%%%%%%%%%%%%%%%%%%%%%

% Estimation of measurement

S = H *p_prd* H.';

%%

switch update
    case 0
        
        for i = 1:11
            S(i,i) = S(i,i) + R(i); %%%%%
        end
        
    case 1
        
        if clock_GPS_pos == 0
            for i = 1:11
                if i == 1 || i == 2
                    S(i,i) = S(i,i) +infinito;
                else
                    S(i,i) = S(i,i) + R(i);
                end
            end
            
        else
            for i = 1:11
                S(i,i) = S(i,i) + R(i); %%%%%
            end
        end
        
    case 2
        
        if clock_GPS_pos == 1 && clock_GPS_vel == 1  && clock_MTi == 1
            
            for i = 1:11
                
                S(i,i) = S(i,i) + R(i);
                
            end
            
        elseif clock_GPS_pos == 0 && clock_GPS_vel == 1 && clock_MTi == 1
            
            for i = 1:11
                if i == 1 || i == 2
                    S(i,i) = S(i,i) +infinito;
                else
                    S(i,i) = S(i,i) + R(i);
                end
            end
            
        elseif clock_GPS_pos == 1 && clock_GPS_vel == 0 && clock_MTi == 1
            
            for i = 1:11
                if i == 4 || i == 5
                    S(i,i) = S(i,i) +infinito;
                else
                    S(i,i) = S(i,i) + R(i);
                end
            end
            
        elseif clock_GPS_pos == 0 && clock_GPS_vel == 0 && clock_MTi == 1
            
            for i = 1:11
                if i == 1 || i == 2 || i == 4 || i == 5
                    S(i,i) = S(i,i) +infinito;
                else
                    S(i,i) = S(i,i) + R(i);
                end
            end
            %
            
            
        elseif clock_GPS_pos == 1 && clock_GPS_vel == 1  && clock_MTi == 0
            
            for i = 1:11
                
                if i == 1 || i == 2 || i == 4 || i == 5 || i == 3
                    
                    S(i,i) = S(i,i) +R(i);
                else
                    S(i,i) = S(i,i) +infinito;
                    
                end
            end
            
        elseif clock_GPS_pos == 0 && clock_GPS_vel == 1 && clock_MTi == 0
            
            for i = 1:11
                
                if i == 4 || i == 5 || i == 3
                    
                    S(i,i) = S(i,i) +R(i);
                else
                    S(i,i) = S(i,i) +infinito;
                    
                end
            end
            
        elseif clock_GPS_pos == 1 && clock_GPS_vel == 0 && clock_MTi == 0
            
            for i = 1:11
                if i == 1 || i == 2 || i == 3
                    
                    S(i,i) = S(i,i) +R(i);
                else
                    S(i,i) = S(i,i) +infinito;
                    
                end
            end
            
        elseif clock_GPS_pos == 0 && clock_GPS_vel == 0 && clock_MTi == 0
            
            for i = 1:11
                if  i == 3
                    S(i,i) = S(i,i) +R(i);
                else
                    S(i,i) = S(i,i) +infinito;
                    
                end
            end
            
        end
end



C = H * p_prd.';

klm_gain = (S \ C).'; %18x11


Z_=zeros(11,1);

Z_(1)= Z(1);  %Pos
Z_(2)= Z(2);
Z_(3)= Z(3);

Z_(4)= Z(4);   %Vel
Z_(5)= Z(5);

Z_(6)= Z(9);   %acc
Z_(7)= Z(10);
Z_(8)= Z(11);

Z_(9)= Z(12);   %vel ang
Z_(10)= Z(13);
Z_(11)= Z(14);

errore_prd = (Z_ - Y_prd); %




residui = errore_prd;

x_est = x_prd + (klm_gain * (errore_prd)).'; %1x18
p_est = p_prd - klm_gain * H * p_prd; %18x18

Cov_est=diag(p_est);

% K_gain=zeros(21,1);
%
% for i=1:21
%
%    K_gain(i)=klm_gain(i,i);
%
% end

%%%%%%%%%%%%%%%%%%%%%%%%
%% linearizzazione dinamica-jacobiano delle equazioni di evoluzione di stato
%%%%%%%%%%%%%%%%%%%%%%%%

F = jac_F_F1B(x_est,a,dt); %18x18

%%%%%%%%%%%%%%%%%
%% aggiornamento con le equazioni della evoluzione di stato %%
%%%%%%%%%%%%%%%%%


x_prd = (f_pred_F1B(x_est,a,dt)).'; %18x1



% Predicted covariance update

p_prd = F * p_est * F.'; %18x18

for k = 1:18
    
    p_prd(k,k) = p_prd(k,k) + Q(k);
    
end

%%%%%%%%%%
%% Exit %%
%%%%%%%%%%

Lat_K = x_est(1);
Long_K = x_est(2);
h_K = x_est(3);

vn_K = x_est(4);
ve_K = x_est(5);
vd_K = x_est(6);


% phi_K = x_est(7);
% theta_K = x_est(8);
% psi_K = x_est(9);

an_K = x_est(7);
ae_K = x_est(8);
ad_K = x_est(9);


p_K = x_est(10);
q_K = x_est(11);
r_K = x_est(12);

baccx = x_est(13);
baccy = x_est(14);
baccz = x_est(15);

bp = x_est(16);
bq = x_est(17);
br = x_est(18);

imbardata = atan2(ve_K,vn_K);
v_K = sqrt(vn_K^2 + ve_K^2);

== matlab function prova_kalman_09_28_BUONO/initializer//Clk_generator 2/Clock Mti/MATLAB Function ==
  data: u input; y output
function y = fcn(u)

y = u(6)|| u(7)|| u(8)||  u(9) || u(10)|| u(11) || u(12) || u(13);

== matlab function prova_kalman_09_28_BUONO/Correzione ingresso1 ==
  data: u input; y output; data input
function y  = fcn(u,data)
%% Correzione ingresso
persistent salto

if isempty(salto)
    salto=0;
end


  if data<0 && u>0 && u-data > pi/2
      
       salto = salto-2*pi;
     
  end
  
  if data>0 && u<0 && data-u > pi/2
      
       salto = salto+2*pi;

  end
  
  y= (u+salto);


  salto_out=salto;

end
%%
